simulink model "ATOM_planning_sim_variable_rear_ratio"  (R2026a)
settings: Solver=ode4  FixedStep=0.01
model workspace (MAT data in the model file):
  vehicle : object (value not decoded)
symbols that are objects in the model workspace (value not decoded): vehicle
undefined symbols (not defined in the file or in its folder): planning_validator, stanley, velocity_smoother
(part 4 of 4)

== matlab function ATOM_planning_sim_variable_rear_ratio/Lateral run()/CalculateStanley /getData/calculate curvature/CalcTrajectoryCurvature ==
  data: trajectory input Bus: TrajectoryDataBus; curvature output; nearest_idx input; idx_dist input
function curvature = ComputeNearestCurvature( ...
    trajectory,...
    nearest_idx, idx_dist)


%% ============================================================
% COMPUTE NEAREST TRAJECTORY CURVATURE
%
% Equivalent to:
%
% autoware::motion_utils::calcTrajectoryCurvatureFrom3Points()
%
% Difference:
%
% - Autoware computes curvature for the whole trajectory
% - Here only the curvature at nearest_idx is required
%   for Stanley controller
%
% Inputs:
%
% trajectory:
%   Reference trajectory
%
% nearest_idx:
%   Nearest trajectory point index
%
% idx_dist:
%   Distance in samples used for three-point fitting
%
%
% Output:
%
% curvature:
%   Local trajectory curvature [1/m]
%
% ============================================================

N = length(trajectory.pose.position.x);



%% Check trajectory length

if N < 3

    curvature = 0;
    return

end



%% Clamp index

nearest_idx = max(1,min(nearest_idx,N));



%% Select three points
%
% Equivalent to Autoware:
%
% p0 = trajectory[i-idx_dist]
% p1 = trajectory[i]
% p2 = trajectory[i+idx_dist]
%
% ============================================================


idx_prev = nearest_idx - min(idx_dist, nearest_idx-1);

idx_next = nearest_idx + min(idx_dist, N-nearest_idx);



p0 = [
    trajectory.pose.position.x(idx_prev),...
    trajectory.pose.position.y(idx_prev)
];


p1 = [
    trajectory.pose.position.x(nearest_idx),...
    trajectory.pose.position.y(nearest_idx)
];


p2 = [
    trajectory.pose.position.x(idx_next),...
    trajectory.pose.position.y(idx_next)
];



%% Compute curvature

curvature = calc_curvature(p0,p1,p2);


end

== matlab function ATOM_planning_sim_variable_rear_ratio/Lateral run()/CalculateStanley /getData/calculate curvature/ComputeIdxDist ==
  data: points_interval input; idx_dist output; vel_smoother input
function idx_dist = ComputeIdxDist( ...
    points_interval, ...
    vel_smoother)

% ComputeIdxDist
%
% Computes the point offset used for trajectory curvature estimation.
%
% The curvature is evaluated using three trajectory points separated by a
% fixed physical distance. Since the trajectory is sampled with a constant
% spatial interval (points_interval), this function converts the desired
% curvature calculation distance into the corresponding point index offset.
%
% In other words, idx_dist represents the number of trajectory points
% corresponding to the specified curvature calculation distance.
%
% Equivalent to the Autoware implementation:
%
% idx_dist = max(int(curvature_calculation_distance / points_interval), 1);

curvature_calculation_distance = vel_smoother(1);

idx_dist = max( ...
    floor(curvature_calculation_distance / points_interval), ...
    1);

== matlab function ATOM_planning_sim_variable_rear_ratio/Lateral run()/CalculateStanley /getData/calculate curvature/ComputePointsInterval ==
  data: input_points_interval input; vel_smoother input; use_resampling input; points_interval output
function points_interval = computePointsInterval(input_points_interval, ...
    vel_smoother, use_resampling)

% Compute the trajectory points interval used for preprocessing.
%
% If resampling is enabled, a constant spatial interval is imposed.
% Otherwise, the original trajectory point spacing is preserved.

sample_ds = vel_smoother(3,1);

if use_resampling

    points_interval = sample_ds;

else

    points_interval = input_points_interval;

end

end

== matlab function ATOM_planning_sim_variable_rear_ratio/Lateral run()/CalculateStanley /VerifyStanleyStatus ==
  data: steering_cmd input; stanley_solved_status output boolean; reason output
function [stanley_solved_status, reason] = VerifyStanleyStatus(steering_cmd)

% reason codes:
% 0 = OK
% 1 = Steering command is NaN/Inf
%
% Attention: in Autoware, reason is a String type. Just Simulink struggles
% with it.

stanley_solved_status = true;
reason = uint8(0);

if ~isfinite(steering_cmd)
    stanley_solved_status = false;
    reason = uint8(1);
end

== matlab function ATOM_planning_sim_variable_rear_ratio/Lateral run()/MATLAB Function1 ==
  data: solved input; previous_status output; reason input; previous_status input; previous_reason input; previous_reason output
function [previous_status, previous_reason] = StanleyStatusManager( ...
    solved,...
    reason,...
    previous_status,...
    previous_reason)

% ATTENTION!!!
% In Autoware, stanley_solved_status (originally mpc_solved_status) 
% is a struct, where equivalently:
% - solved = stanley_solved_status.result
% - reason = stanley_solved_status.reason
%
% StanleyStatusManager here is not implemented since it doesn't change the
% implementation of the controller.

previous_status = solved;
previous_reason = reason;

== matlab function ATOM_planning_sim_variable_rear_ratio/Lateral run()/UpdateSteeringOffset ==
  settings: updateMethod=DISCRETE
  data: steering input; twist input Bus: TwistBus; wheel_base input; update_vel_threshold input; update_steer_threshold input; average_num input; offset_limit input; steering_offset output; veh input
function steering_offset = updateSteeringOffset( ...
    steering,...
    twist,...
    wheel_base,...
    update_vel_threshold,...
    update_steer_threshold,...
    average_num,...
    offset_limit, ...
    veh)


persistent offset_storage
persistent count
persistent current_offset

rear_steering_ratio = veh(29);

if isempty(offset_storage)

    offset_storage = zeros(average_num,1);
    count = 0;
    current_offset = 0;

end


%% Current vehicle state

vx = twist.linear.x;
yaw_rate = twist.angular.z;



%% Check if offset update is allowed

update_offset = ...
    abs(vx) > update_vel_threshold && ...
    abs(steering) < update_steer_threshold;



if update_offset


    %% Estimate steering from vehicle motion

    rear_steering = rear_steering_ratio * steering;

    steer_angle_est = atan( ...
        yaw_rate*wheel_base/vx + tan(rear_steering));



    %% Compute offset

    new_offset = steering - steer_angle_est;



    %% Circular buffer

    count = count + 1;


    if count <= average_num

        offset_storage(count) = new_offset;

    else

        % shift left

        offset_storage(1:end-1)=offset_storage(2:end);

        offset_storage(end)=new_offset;

    end



    %% Compute average

    valid_samples = min(count,average_num);

    current_offset = mean(offset_storage(1:valid_samples));


end



%% Saturation (Autoware getOffset)

steering_offset = min(max(current_offset,...
    -offset_limit),...
    offset_limit);

end

== matlab function ATOM_planning_sim_variable_rear_ratio/Lateral run()/CalculateStanley /calculateFrontSteer - Stanley with variable rear_steering_ratio ==
  data: stanley_data input Bus: StanleyInputDataBus; front_steer output; k_gain input; k_soft input; gain_4WS input; wheelbase input; rear_steer output
function [front_steer, rear_steer] = calculateFrontSteer( ...
    stanley_data,...
    k_gain,...
    k_soft,...
    gain_4WS, ...
    wheelbase)


%% ============================================================
% STANLEY CONTROLLER
%
% Equivalent to the lateral control law used in:
%
% Stanley 4WS:
%
% delta = (yaw_error + atan(k*e_y/(v+k_soft))) * gain_4WS
%
%
% Adaptation for Autoware:
%
% - input data are generated in getDataStanley()
% - reference trajectory is expressed at FRONT AXLE
% - current pose is expressed at FRONT AXLE
% - only front steering command is generated
%
% ============================================================


%% ============================================================
% Extract Stanley data
% ============================================================


lateral_error = stanley_data.lateral_err;

yaw_error = stanley_data.yaw_err;

velocity = stanley_data.front_velocity;

curvature = stanley_data.ref_curvature;



%% ============================================================
% Stanley lateral correction
%
% Equivalent to:
%
% atan(k*e_y/v)
%
% with softening term:
%
% atan(k*e_y/(v+k_soft))
%
% ============================================================


cross_track_term = atan2( ...
    k_gain*(lateral_error),...
    velocity + k_soft);

%% ============================================================
% Steering command
%
% Heading correction + lateral correction
% ============================================================


front_steer = gain_4WS * ((yaw_error + cross_track_term) + atan(curvature*wheelbase));

kappa0 = 0.1;
yaw0 = 0.02;
lat0 = 0.2;
v0 = 15/3.6;

if velocity <= 15/3.6
    kv = 1;
else
    kv = exp(-(velocity-15/3.6)/v0);
end

k = - 0.8 * kv * ...
    (1 - exp(-abs(curvature)/kappa0)) * ...
    (1 - exp(-abs(yaw_error)/yaw0)) * ...
    (1 - exp(-abs(lateral_error)/lat0));

rear_steer = k*front_steer;

end

== matlab function ATOM_planning_sim_variable_rear_ratio/Demanded trajectory generation: smooth Parabola/Smoothed Parabola trajectory ==
  data: x output double; y output double; z output double; qx output double; qy output double; qz output double; qw output double; longitudinal_velocity_mps output double; lateral_velocity_mps output; acceleration_mps2 output; heading_rate_rps output; front_wheel_angle_rad output; rear_wheel_angle_rad output
function [x,y,z,qx,qy,qz,qw,longitudinal_velocity_mps, lateral_velocity_mps, acceleration_mps2, heading_rate_rps, front_wheel_angle_rad, rear_wheel_angle_rad] ...
            = trajectoryGenerator

N=100;

L=50;
Yend=20;


x=zeros(N,1);
y=zeros(N,1);
z=zeros(N,1);


qx=zeros(N,1);
qy=zeros(N,1);
qz=zeros(N,1);
qw=zeros(N,1);

longitudinal_velocity_mps=zeros(N,1);
lateral_velocity_mps=zeros(N,1);
acceleration_mps2=zeros(N,1);
heading_rate_rps=zeros(N,1);
front_wheel_angle_rad=zeros(N,1);
rear_wheel_angle_rad=zeros(N,1);

for i=1:N

    s=(i-1)/(N-1)*L;

    x(i)=s;

    a=Yend/L^2;

    y(i)=a*s^2;

    yaw=atan(2*a*s);


    qx(i)=0;
    qy(i)=0;
    qz(i)=sin(yaw/2);
    qw(i)=cos(yaw/2);


    longitudinal_velocity_mps(i)=5;

end

== matlab function ATOM_planning_sim_variable_rear_ratio/Plot demanded trajectory ==
  data: traj input
function plotTrajectory(traj)

persistent hTraj hArrow


x = traj.pose.position.x;
y = traj.pose.position.y;

yaw = zeros(length(x),1);


for i=1:length(x)

    yaw(i)=2*atan2(...
        traj.pose.orientation.qz(i),...
        traj.pose.orientation.qw(i));

end


if isempty(hTraj)

    figure(2)
    clf
    hold on
    grid on
    axis equal

    hTraj=plot(x,y,'b','LineWidth',2);


    step=5;

    hArrow=quiver(...
        x(1:step:end),...
        y(1:step:end),...
        cos(yaw(1:step:end)),...
        sin(yaw(1:step:end)),...
        0.5,...
        'r');

else

    set(hTraj,...
        'XData',x,...
        'YData',y);

end


drawnow limitrate

end

== matlab function ATOM_planning_sim_variable_rear_ratio/velocity_smoother_node/ApplySteeringRateLimit - velocity_smoother_node/ApplyPreProcess ==
  data: input input Bus: TrajectoryDataBus; use_resempling input boolean; output output Bus: TrajectoryDataBus; points_interval input double
function output = applyPreProcess(input, use_resempling, points_interval)

% ApplyPreProcess
%
% This function reproduces the first stage of Autoware
% SmootherBase::applyPreProcess().
%
% In Autoware, when resampling is enabled, the input trajectory
% is interpolated with a constant spatial interval.
%
% In this Simulink implementation the resampling stage is omitted
% (use_resempling == false)
% The original trajectory points are directly forwarded to the next block.
%

output = input;

end

== matlab function ATOM_planning_sim_variable_rear_ratio/velocity_smoother_node/ApplySteeringRateLimit - velocity_smoother_node/Step1: Calculate curvature assuming the trajectory points interval is constant./CalcTrajectoryCurvature ==
  data: trajectory input Bus: TrajectoryDataBus; curvature output; idx_dist input
function curvature = ComputeTrajectoryCurvature( ...
    trajectory, ...
    idx_dist)

% ComputeTrajectoryCurvature
%
% Computes the geometric curvature of a trajectory using a three-point
% circle fitting method.
%
% This function reproduces the behavior of:
%
% autoware_motion_utils::calcTrajectoryCurvatureFrom3Points()
%
% used inside:
%
% autoware_velocity_smoother
%
% In the original Autoware implementation, the curvature computation:
%
%   curvature = calc_curvature(p0,p1,p2)
%
% is protected by a C++ try/catch block. If the circle fitting fails
% (for example due to degenerate geometry), Autoware keeps the previous
% curvature value.
%
% MATLAB/Simulink code generation does not support try/catch constructs.
% Therefore this implementation assumes that calc_curvature() is robust
% and handles degenerate cases internally.
%
% Inputs
% -------
% trajectory : struct
%
%   MATLAB representation of Autoware TrajectoryPoints.
%
%   Autoware source:
%
%   autoware_motion_utils/src/trajectory/conversion.cpp
%
%   converts:
%
%       autoware_planning_msgs::msg::Trajectory
%
%   into:
%
%       std::vector<autoware_planning_msgs::msg::TrajectoryPoint>
%
%   via:
%
    % std::vector<autoware_planning_msgs::msg::TrajectoryPoint> convertToTrajectoryPointArray(
    % const autoware_planning_msgs::msg::Trajectory & trajectory)
    % {
    %     std::vector<autoware_planning_msgs::msg::TrajectoryPoint> output(trajectory.points.size());
    %     std::copy(trajectory.points.begin(), trajectory.points.end(), output.begin());
    %     return output;
    % }
%
%
%
%   Each trajectory point contains:
%
%       geometry_msgs/msg/Point pose.position
%
%   with:
%
%       x, y, z
%
%   MATLAB representation:
%
%       trajectory.pose.position.x
%       trajectory.pose.position.y
%       trajectory.pose.position.z
%
%
% idx_dist : scalar
%
%   Number of trajectory samples used as offset for the three-point
%   curvature estimation.
%
%   In Autoware:
%
%       idx_dist =
%       max(floor(curvature_calculation_distance / points_interval),1)
%
%
% Output
% -------
% curvature : Nx1 vector
%
%   Estimated trajectory curvature [1/m].

num_points = length(trajectory.pose.position.x);


%% Not enough trajectory points

% Autoware:
%
% if (trajectory.size() < 3)
% {
%     return vector filled with zeros;
% }

if num_points < 3
    curvature = zeros(num_points,1);
    return;
end


%% Limit idx_dist according to trajectory size

% Autoware:
%
% max_idx_dist =
% floor((trajectory.size()-1)/2)
%
% idx_dist =
% max(1,min(idx_dist,max_idx_dist))

max_idx_dist = floor((num_points-1)/2);

idx_dist = max(1,min(idx_dist,max_idx_dist));


%% Initialize curvature vector

% Autoware:
%
% std::vector<double> k_arr(trajectory.size(),0.0);

curvature = zeros(num_points,1);


%% Three-point curvature estimation

% Autoware:
%
% for (size_t i = 1; i + 1 < trajectory.size(); i++)

% MATLAB indexing:
%
% i = 2 ... N-1

for i = 2:num_points-1


    % Select the three points:
    %
    % p0 : idx_dist samples before
    % p1 : current trajectory point
    % p2 : idx_dist samples after
    %
    % Equivalent to Autoware:
    %
    % p0 = get_point(
    %       trajectory.at(i - min(idx_dist,i)))
    %
    % p1 = get_point(
    %       trajectory.at(i))
    %
    % p2 = get_point(
    %       trajectory.at(
    %       i + min(idx_dist,size-i-1)))


    idx_prev = i - min(idx_dist,i-1);

    idx_curr = i;

    idx_next = i + min(idx_dist,num_points-i);


    % geometry_msgs/msg/Point:
    %
    % float64 x
    % float64 y
    % float64 z

    p0 = [
        trajectory.pose.position.x(idx_prev), ...
        trajectory.pose.position.y(idx_prev), ...
        trajectory.pose.position.z(idx_prev)
        ];

    p1 = [
        trajectory.pose.position.x(idx_curr), ...
        trajectory.pose.position.y(idx_curr), ...
        trajectory.pose.position.z(idx_curr)
        ];

    p2 = [
        trajectory.pose.position.x(idx_next), ...
        trajectory.pose.position.y(idx_next), ...
        trajectory.pose.position.z(idx_next)
        ];


    %% Compute curvature

    % Autoware:
    %
    % try
    % {
    %     curvature = calc_curvature(p0,p1,p2);
    % }
    %
    % catch(...)
    % {
    %     curvature = previous curvature;
    % }
    %
    % try/catch removed because unsupported by Simulink Coder.

    curvature(i) = calc_curvature(p0,p1,p2);


end


%% Boundary curvature completion

% Autoware:
%
% k_arr.at(0) = k_arr.at(1);
% k_arr.back() = k_arr.at(size-2);

curvature(1) = curvature(2);

curvature(end) = curvature(end-1);


end
